simulink model "DcMotorSpeedControlSimulink"  (R2019b)
settings: Solver=VariableStepAuto  StartTime=0.0  StopTime=1.0  RelTol=1e-3
values from neighbouring files (symbols this model uses):
  b = 0.1    [DcMotorSpeedControl.m]
  J = 0.01    [DcMotorSpeedControl.m]
  K = 0.01    [DcMotorSpeedControl.m]
  L = 0.5    [DcMotorSpeedControl.m]
  R = 1    [DcMotorSpeedControl.m]
settings Model: Creator=fhasan1  LastModifiedBy=fhasan1

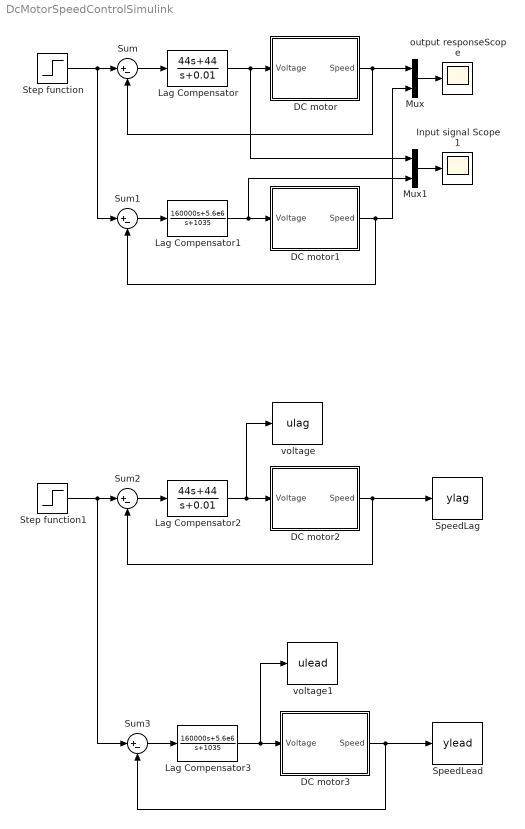
== system DcMotorSpeedControlSimulink ==
  DC motor : Subsystem
  DC motor1 : Subsystem
  DC motor2 : Subsystem
  DC motor3 : Subsystem
  Input signal Scope 1 : Scope
  Lag Compensator : TransferFcn  Numerator=[44 44 ]  Denominator=[1 0.01 ]
  Lag Compensator1 : TransferFcn  Numerator=[160000 5.6e6 ]  Denominator=[1 1035 ]
  Lag Compensator2 : TransferFcn  Numerator=[44 44 ]  Denominator=[1 0.01 ]
  Lag Compensator3 : TransferFcn  Numerator=[160000 5.6e6 ]  Denominator=[1 1035 ]
  Mux : Mux  Inputs=2
  Mux1 : Mux  Inputs=2
  SpeedLag : ToWorkspace  VariableName=ylag  SampleTime=-1
      settings: Save2DSignal=2-D array (concatenate along first dimension)
  SpeedLead : ToWorkspace  VariableName=ylead  SampleTime=-1
      settings: Save2DSignal=2-D array (concatenate along first dimension)
  Step function : Step  Time=0  SampleTime=0
  Step function1 : Step  Time=0  SampleTime=0
  Sum{,1..3} (4 alike) : Sum  Inputs=|+-
  "output responseScope " : Scope
  voltage : ToWorkspace  VariableName=ulag  SampleTime=-1
      settings: Save2DSignal=2-D array (concatenate along first dimension)
  voltage1 : ToWorkspace  VariableName=ulead  SampleTime=-1
      settings: Save2DSignal=2-D array (concatenate along first dimension)
  wires:
  DC motor/1(Speed) -> Mux/1, Sum/2
  Sum/1 -> Lag Compensator/1
  Lag Compensator/1 -> Mux1/1, DC motor/1(Voltage)
  DC motor1/1(Speed) -> Mux/2, Sum1/2
  Sum1/1 -> Lag Compensator1/1
  Lag Compensator1/1 -> Mux1/2, DC motor1/1(Voltage)
  Mux/1 -> "output responseScope "/1
  Step function/1 -> Sum1/1, Sum/1
  Sum3/1 -> Lag Compensator3/1
  Lag Compensator3/1 -> voltage1/1, DC motor3/1(Voltage)
  DC motor3/1(Speed) -> SpeedLead/1, Sum3/2
  DC motor2/1(Speed) -> SpeedLag/1, Sum2/2
  Sum2/1 -> Lag Compensator2/1
  Lag Compensator2/1 -> voltage/1, DC motor2/1(Voltage)
  Step function1/1 -> Sum3/1, Sum2/1
  Mux1/1 -> Input signal Scope 1/1

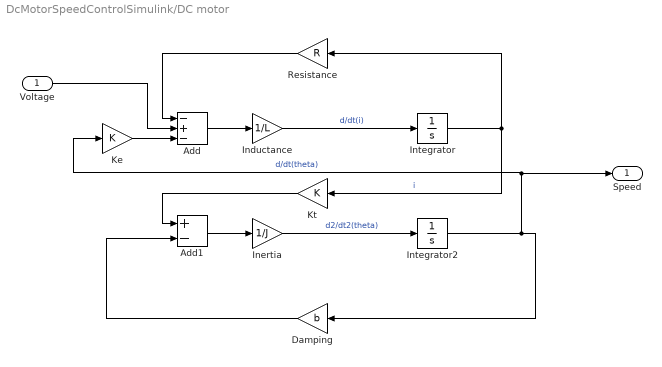
== system DcMotorSpeedControlSimulink/DC motor ==
  Voltage : Inport
  Add : Sum  Inputs=-+-
  Add1 : Sum  Inputs=+-
  Damping : Gain  Gain=b
  Inductance : Gain  Gain=1/L
  Inertia : Gain  Gain=1/J
  Integrator : Integrator
  Integrator2 : Integrator
  Ke : Gain  Gain=K
  Kt : Gain  Gain=K
  Resistance : Gain  Gain=R
  Speed : Outport
  wires:
  Integrator2/1 -> Speed/1, Ke/1, Damping/1  "d/dt(theta)"
  Add/1 -> Inductance/1
  Kt/1 -> Add1/1
  Damping/1 -> Add1/2
  Add1/1 -> Inertia/1
  Integrator/1 -> Resistance/1, Kt/1  "i"
  Inductance/1 -> Integrator/1  "d/dt(i)"
  Resistance/1 -> Add/1
  Inertia/1 -> Integrator2/1  "d2/dt2(theta)"
  Voltage/1 -> Add/2
  Ke/1 -> Add/3

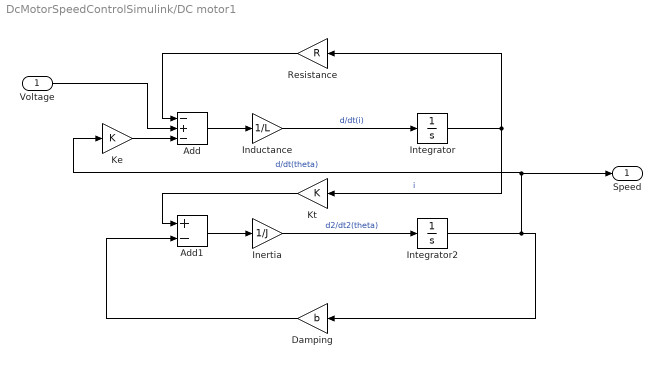
== system DcMotorSpeedControlSimulink/DC motor1 ==
  Voltage : Inport
  Add : Sum  Inputs=-+-
  Add1 : Sum  Inputs=+-
  Damping : Gain  Gain=b
  Inductance : Gain  Gain=1/L
  Inertia : Gain  Gain=1/J
  Integrator : Integrator
  Integrator2 : Integrator
  Ke : Gain  Gain=K
  Kt : Gain  Gain=K
  Resistance : Gain  Gain=R
  Speed : Outport
  wires:
  Integrator2/1 -> Speed/1, Ke/1, Damping/1  "d/dt(theta)"
  Add/1 -> Inductance/1
  Kt/1 -> Add1/1
  Damping/1 -> Add1/2
  Add1/1 -> Inertia/1
  Integrator/1 -> Resistance/1, Kt/1  "i"
  Inductance/1 -> Integrator/1  "d/dt(i)"
  Resistance/1 -> Add/1
  Inertia/1 -> Integrator2/1  "d2/dt2(theta)"
  Voltage/1 -> Add/2
  Ke/1 -> Add/3

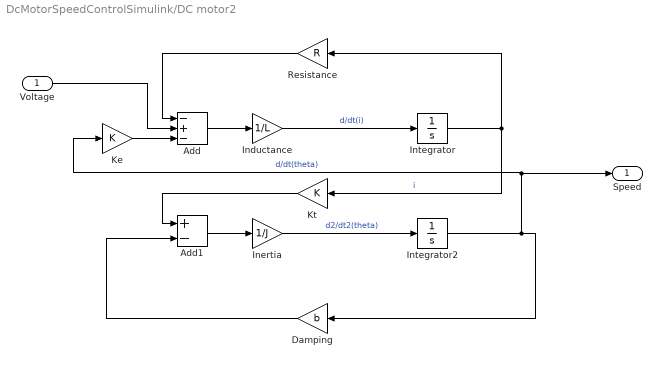
== system DcMotorSpeedControlSimulink/DC motor2 ==
  Voltage : Inport
  Add : Sum  Inputs=-+-
  Add1 : Sum  Inputs=+-
  Damping : Gain  Gain=b
  Inductance : Gain  Gain=1/L
  Inertia : Gain  Gain=1/J
  Integrator : Integrator
  Integrator2 : Integrator
  Ke : Gain  Gain=K
  Kt : Gain  Gain=K
  Resistance : Gain  Gain=R
  Speed : Outport
  wires:
  Integrator2/1 -> Speed/1, Ke/1, Damping/1  "d/dt(theta)"
  Add/1 -> Inductance/1
  Kt/1 -> Add1/1
  Damping/1 -> Add1/2
  Add1/1 -> Inertia/1
  Integrator/1 -> Resistance/1, Kt/1  "i"
  Inductance/1 -> Integrator/1  "d/dt(i)"
  Resistance/1 -> Add/1
  Inertia/1 -> Integrator2/1  "d2/dt2(theta)"
  Voltage/1 -> Add/2
  Ke/1 -> Add/3

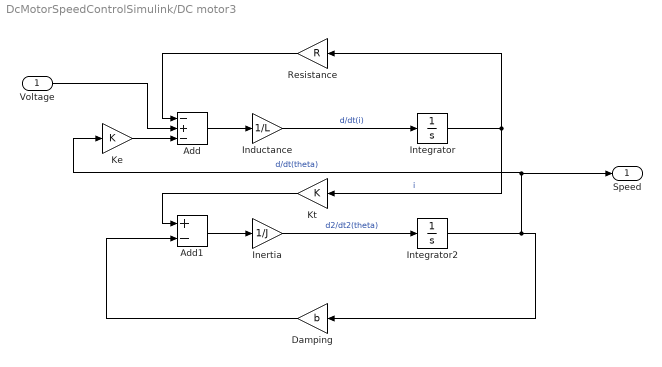
== system DcMotorSpeedControlSimulink/DC motor3 ==
  Voltage : Inport
  Add : Sum  Inputs=-+-
  Add1 : Sum  Inputs=+-
  Damping : Gain  Gain=b
  Inductance : Gain  Gain=1/L
  Inertia : Gain  Gain=1/J
  Integrator : Integrator
  Integrator2 : Integrator
  Ke : Gain  Gain=K
  Kt : Gain  Gain=K
  Resistance : Gain  Gain=R
  Speed : Outport
  wires:
  Integrator2/1 -> Speed/1, Ke/1, Damping/1  "d/dt(theta)"
  Add/1 -> Inductance/1
  Kt/1 -> Add1/1
  Damping/1 -> Add1/2
  Add1/1 -> Inertia/1
  Integrator/1 -> Resistance/1, Kt/1  "i"
  Inductance/1 -> Integrator/1  "d/dt(i)"
  Resistance/1 -> Add/1
  Inertia/1 -> Integrator2/1  "d2/dt2(theta)"
  Voltage/1 -> Add/2
  Ke/1 -> Add/3
